simulink model "TwoTankOpenLoop"  (R2016a)
settings: Solver=ode45  StartTime=0.0  StopTime=1000  MaxStep=0.2  RelTol=1e-3
model workspace (MAT data in the model file):
  TwoTankOPTrim : opcond.OperatingReport (value not decoded)
  op_trim1 : opcond.OperatingReport (value not decoded)
  op_trim3 : opcond.OperatingReport (value not decoded)
undefined symbols (not defined in the file): Initials, inputOpt, kl, L1i, T1i, timeDelay
libraries: simulink x1, TTLibrary x1
settings Model: Creator=blindner  LastModifiedBy=blindner
settings DataIOCC: ExternalInput=getinputstruct(op_trim1)  InitialState=getstatestruct(op_trim1)  SaveFormat=Array  SaveOutput=off  SaveTime=off
settings DebuggingCC: SolverPrmCheckMsg=warning
settings HardwareCC: ProdBitPerPointer=32  ProdLargestAtomicFloat=None  ProdIntDivRoundTo=Undefined  ProdEndianess=Unspecified  ProdWordSize=32  ProdHWDeviceType=32-bit Generic
settings ModelReferenceCC: PropagateSignalLabelsOutOfModel=off
settings ConfigComp: CovModelRefEnable=Off  CovSFcnEnable=off

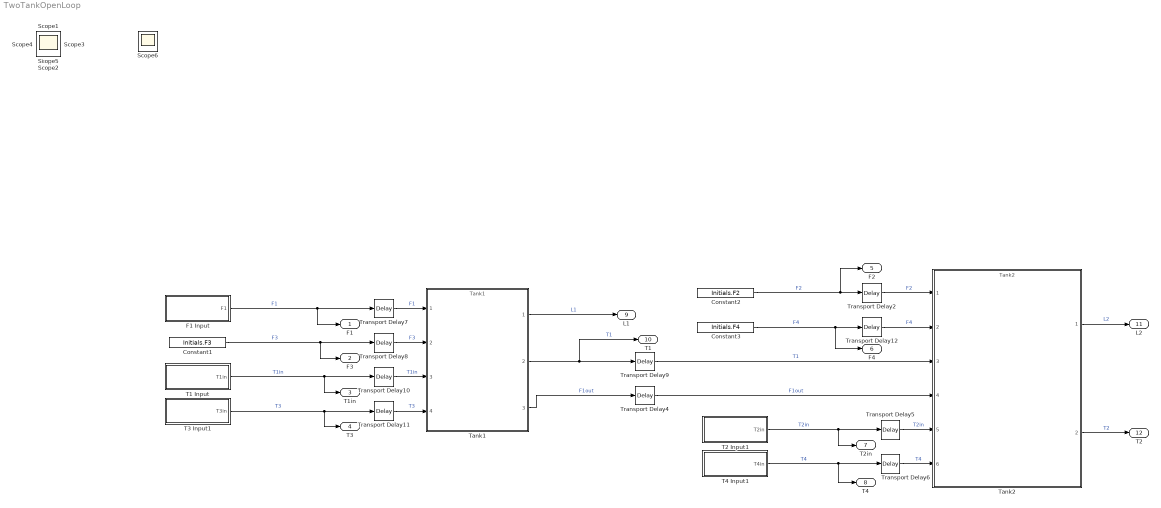
== system TwoTankOpenLoop ==
  Constant1 : Constant  Value=Initials.F3
  Constant2 : Constant  Value=Initials.F2
  Constant3 : Constant  Value=Initials.F4
  F1 Input : Subsystem  Variant=on
  T1 Input : Subsystem  Variant=on
  T2 Input1 : Subsystem  Variant=on
  T3 Input1 : Subsystem  Variant=on
  T4 Input1 : Subsystem  Variant=on
  Tank1 : ModelReference  ModelNameDialog=Tank1  SimulationMode=Normal  ModelReferenceVersion=1.161
  Tank2 : ModelReference  ModelNameDialog=Tank2  SimulationMode=Normal  ModelReferenceVersion=1.153
  Transport Delay10 : TransportDelay  DelayTime=timeDelay.F1  InitialOutput=inputOpt.T1in.start  TransDelayFeedthrough=on
  Transport Delay11 : TransportDelay  DelayTime=timeDelay.F3  InitialOutput=inputOpt.T3.start  TransDelayFeedthrough=on
  Transport Delay12 : TransportDelay  DelayTime=timeDelay.F4  InitialOutput=Initials.F4  TransDelayFeedthrough=on
  Transport Delay2 : TransportDelay  DelayTime=timeDelay.F2  InitialOutput=Initials.F2  TransDelayFeedthrough=on
  Transport Delay4 : TransportDelay  DelayTime=timeDelay.F1Out  InitialOutput=(L1i)^0.5*kl  TransDelayFeedthrough=on
  Transport Delay5 : TransportDelay  DelayTime=timeDelay.F2  InitialOutput=inputOpt.T2in.start  TransDelayFeedthrough=on
  Transport Delay6 : TransportDelay  DelayTime=timeDelay.F4  InitialOutput=inputOpt.T4.start  TransDelayFeedthrough=on
  Transport Delay7 : TransportDelay  DelayTime=timeDelay.F1  InitialOutput=Initials.F1  TransDelayFeedthrough=on
  Transport Delay8 : TransportDelay  DelayTime=timeDelay.F3  InitialOutput=Initials.F3  TransDelayFeedthrough=on
  Transport Delay9 : TransportDelay  DelayTime=timeDelay.F1Out  InitialOutput=T1i  TransDelayFeedthrough=on
  F1 : Outport
  F3 : Outport  Port=2
  T1in : Outport  Port=3
  T3 : Outport  Port=4
  F2 : Outport  Port=5
  F4 : Outport  Port=6
  T2in : Outport  Port=7
  T4 : Outport  Port=8
  L1 : Outport  Port=9  OutDataTypeStr=double  PortDimensions=1
  T1 : Outport  Port=10  OutDataTypeStr=double  PortDimensions=1
  L2 : Outport  Port=11  OutDataTypeStr=double  PortDimensions=1
  T2 : Outport  Port=12  OutDataTypeStr=double  PortDimensions=1
  Scope{,1..6} (7 alike) : Scope
  wires:
  T1 Input/1(T1in) -> T1in/1, Transport Delay10/1  "T1in"
  T3 Input1/1(T3in) -> T3/1, Transport Delay11/1  "T3"
  F1 Input/1(F1) -> F1/1, Transport Delay7/1  "F1"
  Constant1/1 -> F3/1, Transport Delay8/1  "F3"
  Constant2/1 -> F2/1, Transport Delay2/1  "F2"
  Constant3/1 -> F4/1, Transport Delay12/1  "F4"
  T4 Input1/1(T4in) -> T4/1, Transport Delay6/1  "T4"
  T2 Input1/1(T2in) -> T2in/1, Transport Delay5/1  "T2in"
  Transport Delay5/1 -> Tank2/5  "T2in"
  Transport Delay6/1 -> Tank2/6  "T4"
  Transport Delay7/1 -> Tank1/1  "F1"
  Transport Delay8/1 -> Tank1/2  "F3"
  Transport Delay10/1 -> Tank1/3  "T1in"
  Transport Delay11/1 -> Tank1/4  "T3"
  Transport Delay2/1 -> Tank2/1  "F2"
  Transport Delay12/1 -> Tank2/2  "F4"
  Transport Delay4/1 -> Tank2/4  "F1out"
  Transport Delay9/1 -> Tank2/3  "T1"
  Tank1/3 -> Transport Delay4/1  "F1out"
  Tank1/2 -> T1/1, Transport Delay9/1  "T1"
  Tank1/1 -> L1/1  "L1"
  Tank2/1 -> L2/1  "L2"
  Tank2/2 -> T2/1  "T2"

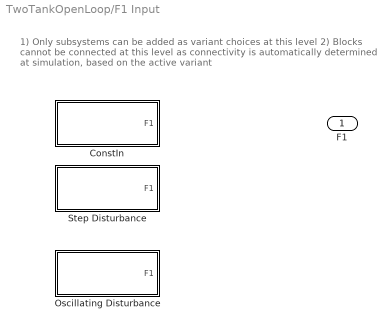
== system TwoTankOpenLoop/F1 Input ==
  note: 1) Only subsystems can be added as variant choices at this level
      | 2) Blocks cannot be connected at this level as connectivity is
      | automatically determined at simulation, based on the active variant
  ConstIn : Subsystem  VariantControl=(default)
  Oscillating Disturbance : Subsystem  VariantControl=F1Oscillating
  Step Disturbance : Subsystem  VariantControl=F1Step
  F1 : Outport

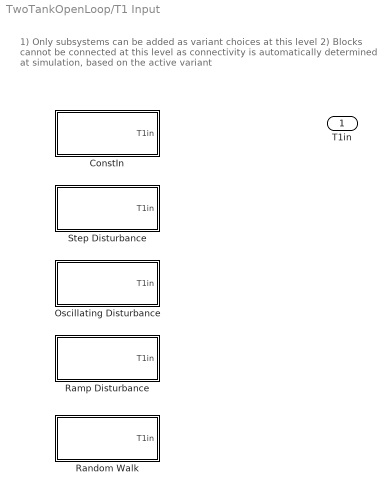
== system TwoTankOpenLoop/T1 Input ==
  note: 1) Only subsystems can be added as variant choices at this level
      | 2) Blocks cannot be connected at this level as connectivity is
      | automatically determined at simulation, based on the active variant
  ConstIn : Subsystem  VariantControl=(default)
  Oscillating Disturbance : Subsystem  VariantControl=T1Oscillating
  Ramp Disturbance : Subsystem  VariantControl=T1Ramp
  Random Walk : Subsystem  VariantControl=T1RW
  Step Disturbance : Subsystem  VariantControl=T1Step
  T1in : Outport

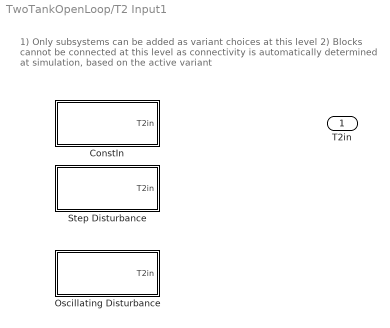
== system TwoTankOpenLoop/T2 Input1 ==
  note: 1) Only subsystems can be added as variant choices at this level
      | 2) Blocks cannot be connected at this level as connectivity is
      | automatically determined at simulation, based on the active variant
  ConstIn : Subsystem  VariantControl=(default)
  Oscillating Disturbance : Subsystem  VariantControl=T2Oscillating
  Step Disturbance : Subsystem  VariantControl=T2Step
  T2in : Outport

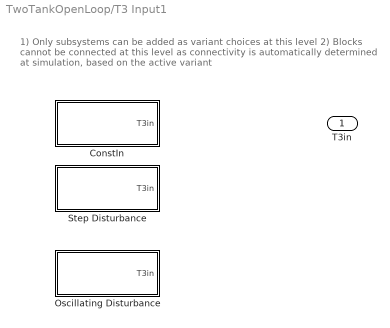
== system TwoTankOpenLoop/T3 Input1 ==
  note: 1) Only subsystems can be added as variant choices at this level
      | 2) Blocks cannot be connected at this level as connectivity is
      | automatically determined at simulation, based on the active variant
  ConstIn : Subsystem  VariantControl=(default)
  Oscillating Disturbance : Subsystem  VariantControl=T3Oscillating
  Step Disturbance : Subsystem  VariantControl=T3Step
  T3in : Outport

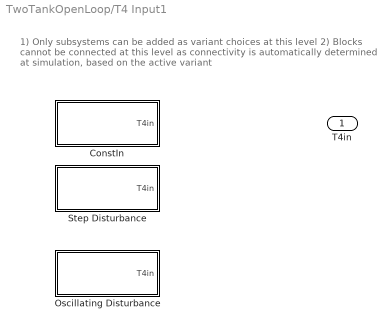
== system TwoTankOpenLoop/T4 Input1 ==
  note: 1) Only subsystems can be added as variant choices at this level
      | 2) Blocks cannot be connected at this level as connectivity is
      | automatically determined at simulation, based on the active variant
  ConstIn : Subsystem  VariantControl=(default)
  Oscillating Disturbance : Subsystem  VariantControl=T4Oscillating
  Step Disturbance : Subsystem  VariantControl=T4Step
  T4in : Outport

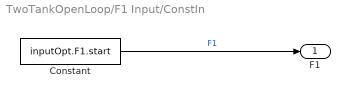
== system TwoTankOpenLoop/F1 Input/ConstIn ==
  Constant : Constant  Value=inputOpt.F1.start
  F1 : Outport
  wires:
  Constant/1 -> F1/1  "F1"

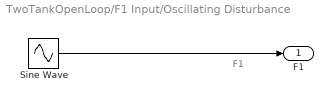
== system TwoTankOpenLoop/F1 Input/Oscillating Disturbance ==
  note: F1
  Sine Wave : Sin  Amplitude=inputOpt.F1.amplitude  Bias=inputOpt.F1.start  Frequency=pi/inputOpt.F1.period  SampleTime=0
  F1 : Outport
  wires:
  Sine Wave/1 -> F1/1

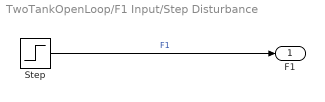
== system TwoTankOpenLoop/F1 Input/Step Disturbance ==
  Step : Step  Time=inputOpt.F1.time  Before=inputOpt.F1.start  After=inputOpt.F1.end  SampleTime=0
  F1 : Outport
  wires:
  Step/1 -> F1/1  "F1"

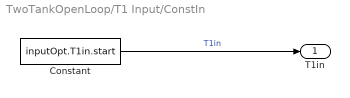
== system TwoTankOpenLoop/T1 Input/ConstIn ==
  Constant : Constant  Value=inputOpt.T1in.start
  T1in : Outport
  wires:
  Constant/1 -> T1in/1  "T1in"

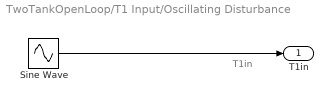
== system TwoTankOpenLoop/T1 Input/Oscillating Disturbance ==
  note: T1in
  Sine Wave : Sin  Amplitude=inputOpt.T1in.amplitude  Bias=inputOpt.T1in.start  Frequency=pi/inputOpt.T1in.period  SampleTime=0
  T1in : Outport
  wires:
  Sine Wave/1 -> T1in/1

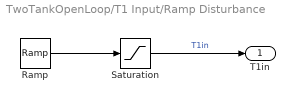
== system TwoTankOpenLoop/T1 Input/Ramp Disturbance ==
  Ramp : simulink/Sources/Ramp  slope=(inputOpt.T1in.end-inputOpt.T1in.start)/inputOpt.T1in.period  start=inputOpt.T1in.time  X0=inputOpt.T1in.start
  Saturation : Saturate  UpperLimit=inputOpt.T1in.end  LowerLimit=-inf
  T1in : Outport
  wires:
  Saturation/1 -> T1in/1  "T1in"
  Ramp/1 -> Saturation/1

== system TwoTankOpenLoop/T1 Input/Random Walk ==
  random walk1 : TTLibrary/random walk  addNoise=1  noiseSeed=randi(1000)  sampleTime=inputOpt.sampleTime  grad=0.5  IC=0  UB=inf  LB=-inf
  T1in : Outport
  wires:
  random walk1/1 -> T1in/1  "T1in"

== system TwoTankOpenLoop/T1 Input/Step Disturbance ==
  Step : Step  Time=inputOpt.T1in.time  Before=inputOpt.T1in.start  After=inputOpt.T1in.end  SampleTime=0
  T1in : Outport
  wires:
  Step/1 -> T1in/1  "T1in"

== system TwoTankOpenLoop/T2 Input1/ConstIn ==
  Constant : Constant  Value=inputOpt.T2in.start
  T2in : Outport
  wires:
  Constant/1 -> T2in/1  "T2in"

== system TwoTankOpenLoop/T2 Input1/Oscillating Disturbance ==
  note: T2in
  Sine Wave : Sin  Amplitude=inputOpt.T2in.amplitude  Bias=inputOpt.T2in.start  Frequency=pi/inputOpt.T2in.period  SampleTime=0
  T2in : Outport
  wires:
  Sine Wave/1 -> T2in/1

== system TwoTankOpenLoop/T2 Input1/Step Disturbance ==
  Step : Step  Time=inputOpt.T2in.time  Before=inputOpt.T2in.start  After=inputOpt.T2in.end  SampleTime=0
  T2in : Outport
  wires:
  Step/1 -> T2in/1  "T2in"

== system TwoTankOpenLoop/T3 Input1/ConstIn ==
  Constant : Constant  Value=inputOpt.T3.start
  T3in : Outport
  wires:
  Constant/1 -> T3in/1  "T3in"

== system TwoTankOpenLoop/T3 Input1/Oscillating Disturbance ==
  note: T3in
  Sine Wave : Sin  Amplitude=inputOpt.T3.amplitude  Bias=inputOpt.T3.start  Frequency=pi/inputOpt.T3.period  SampleTime=0
  T3in : Outport
  wires:
  Sine Wave/1 -> T3in/1

== system TwoTankOpenLoop/T3 Input1/Step Disturbance ==
  Step : Step  Time=inputOpt.T3.time  Before=inputOpt.T3.start  After=inputOpt.T3.end  SampleTime=0
  T3in : Outport
  wires:
  Step/1 -> T3in/1  "T3in"

== system TwoTankOpenLoop/T4 Input1/ConstIn ==
  Constant : Constant  Value=inputOpt.T4.start
  T4in : Outport
  wires:
  Constant/1 -> T4in/1  "T3in"

== system TwoTankOpenLoop/T4 Input1/Oscillating Disturbance ==
  note: T4in
  Sine Wave : Sin  Amplitude=inputOpt.T4.amplitude  Bias=inputOpt.T4.start  Frequency=pi/inputOpt.T2in.period  SampleTime=0
  T4in : Outport
  wires:
  Sine Wave/1 -> T4in/1

== system TwoTankOpenLoop/T4 Input1/Step Disturbance ==
  Step : Step  Time=inputOpt.T4.time  Before=inputOpt.T4.start  After=inputOpt.T4.end  SampleTime=0
  T4in : Outport
  wires:
  Step/1 -> T4in/1  "T4in"
